simulink model "Model2018a"  (R2018a)
settings: Solver=FixedStepAuto  StartTime=t0  StopTime=tk  FixedStep=ts  RelTol=1e-3
values from neighbouring files (symbols this model uses):
  c1 = 0.2    [Wywolawczy.m]    (also in Wywolawczy2.m; Wywolawczy3.m; Wywolawczy4.m; Wywolawczy5.m)
  c2 = 1    [Wywolawczy.m]    (also in Wywolawczy2.m; Wywolawczy3.m; Wywolawczy4.m; Wywolawczy5.m)
  k1 = 2    [Wywolawczy.m]    (also in Wywolawczy2.m; Wywolawczy3.m; Wywolawczy4.m; Wywolawczy5.m)
  k2 = 2    [Wywolawczy.m]    (also in Wywolawczy2.m; Wywolawczy3.m; Wywolawczy4.m; Wywolawczy5.m)
  m1 = 3    [Wywolawczy.m]    (also in Wywolawczy2.m; Wywolawczy3.m; Wywolawczy4.m; Wywolawczy5.m)
  m2 = 0.5    [Wywolawczy.m]    (also in Wywolawczy2.m; Wywolawczy3.m; Wywolawczy4.m; Wywolawczy5.m)
  ts = 1e-2    (= 0.01)    [Wywolawczy.m]    (also in Wywolawczy2.m; Wywolawczy3.m; Wywolawczy4.m; Wywolawczy5.m)
undefined symbols (not defined in the file or in its folder): DiscIntNeverNeededParam
settings Model: Creator=user  LastModifiedBy=user
settings DebuggingCC: LibraryContextMissingDiagnostic=warning
settings SFSimCC: SimUseLocalCustomCode=on
settings RTWCC: RTWUseLocalCustomCode=on

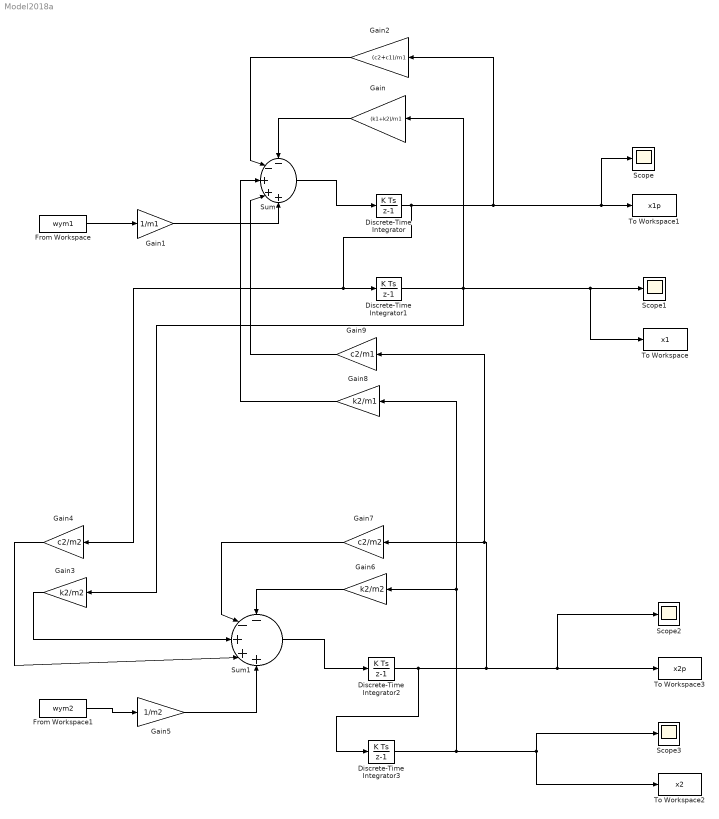
== system Model2018a ==
  Discrete-Time Integrator{,1..3} (4 alike) : DiscreteIntegrator  SampleTime=-1  ICPrevOutput=DiscIntNeverNeededParam  ICPrevScaledInput=DiscIntNeverNeededParam
  From Workspace : FromWorkspace  VariableName=wym1  SampleTime=ts
  From Workspace1 : FromWorkspace  VariableName=wym2  SampleTime=ts
  Gain : Gain  Gain=(k1+k2)/m1
  Gain1 : Gain  Gain=1/m1
  Gain2 : Gain  Gain=(c2+c1)/m1
  Gain3 : Gain  Gain=k2/m2
  Gain4 : Gain  Gain=c2/m2
  Gain5 : Gain  Gain=1/m2
  Gain6 : Gain  Gain=k2/m2
  Gain7 : Gain  Gain=c2/m2
  Gain8 : Gain  Gain=k2/m1
  Gain9 : Gain  Gain=c2/m1
  Scope{,1..3} (4 alike) : Scope
  Sum : Sum  Inputs=--+++
  Sum1 : Sum  Inputs=--+++
  To Workspace : ToWorkspace  VariableName=x1  SampleTime=-1
      settings: Save2DSignal=2-D array (concatenate along first dimension)
  To Workspace1 : ToWorkspace  VariableName=x1p  SampleTime=-1
      settings: Save2DSignal=2-D array (concatenate along first dimension)
  To Workspace2 : ToWorkspace  VariableName=x2  SampleTime=-1
      settings: Save2DSignal=2-D array (concatenate along first dimension)
  To Workspace3 : ToWorkspace  VariableName=x2p  SampleTime=-1
      settings: Save2DSignal=2-D array (concatenate along first dimension)
  wires:
  From Workspace/1 -> Gain1/1
  Gain/1 -> Sum/1
  Gain2/1 -> Sum/2
  Sum/1 -> Discrete-Time Integrator/1
  Discrete-Time Integrator/1 -> Gain4/1, Discrete-Time Integrator1/1, Gain2/1, To Workspace1/1, Scope/1
  Discrete-Time Integrator1/1 -> Gain3/1, Gain/1, To Workspace/1, Scope1/1
  Gain1/1 -> Sum/5
  Sum1/1 -> Discrete-Time Integrator2/1
  Discrete-Time Integrator2/1 -> Discrete-Time Integrator3/1, Gain9/1, Gain7/1, Scope2/1, To Workspace3/1
  Discrete-Time Integrator3/1 -> Gain8/1, Gain6/1, To Workspace2/1, Scope3/1
  From Workspace1/1 -> Gain5/1
  Gain5/1 -> Sum1/5
  Gain7/1 -> Sum1/2
  Gain3/1 -> Sum1/3
  Gain4/1 -> Sum1/4
  Gain6/1 -> Sum1/1
  Gain9/1 -> Sum/4
  Gain8/1 -> Sum/3
